simulink model "controller_ballcatcher_overdo"  (R2018b)
settings: Solver=FixedStepDiscrete  StartTime=0.0  StopTime=10.0  FixedStep=param_controller.T_a  RelTol=1e-3
InitFcn:
  | iiwa_joint_trajectoryfollowingcontrol_rigid_parameters;
values from neighbouring files (symbols this model uses):
  estimator_init_struct = struct()    [init_estimator_struct.m]
  filter_tau_p_slow_T_1 = filter_tau_slow_T_1    [parameters.m]
  filter_tau_p_T_1 = filter_tau_T_1    [parameters.m]
  filter_tau_slow_T_1 = 1./(2*pi*[200;200;200;200;200;200;200])    [parameters.m]
  filter_tau_T_1 = 1./(2*pi*[400;400;400;400;500;1000;1000])    [parameters.m]
  filter_theta_p_slow_T_1 = filter_tau_slow_T_1    [parameters.m]
  filter_theta_p_T_1 = filter_tau_T_1    [parameters.m]
  filter_theta_slow_T_1 = filter_tau_slow_T_1    [parameters.m]
  height_of_catch = 0.9    [init_estimator_struct.m]
  optitrack_data = struct()    [init_parabola.m]
  param_nullspace = struct()    [parameters.m]
  param_robot = struct()    [parameters.m]
  positions = struct()    [init_common_positions.m]
  sensor_torque_offset = [0.53;-0.095;-0.189;0.07;-0.058;0.0025;-0.12]    [parameters.m]
  timing = struct()    [parameters.m]
undefined symbols (not defined in the file or in its folder): param_controller
libraries: simulink_extras x1
(part 2 of 2)

== matlab function controller_ballcatcher_overdo/Chart1/estimate_parabola/Parabola Estimator ==
  data: t_in input; t_start input; point_in input; height_of_catch parameter; pd output; estimator_init_struct parameter; init input; pd_p output; use_pred output; t_catch_predict output; timing parameter; prediction_update output; init_number_of_samples input
function [pd,pd_p,use_pred,t_catch_predict,prediction_update] = fcn(t_in,t_start,point_in,height_of_catch,estimator_init_struct,init,timing,init_number_of_samples)

    t_for_est = t_in-t_start;
    t_move_start = timing.T_optitrack*init_number_of_samples;
    t_start_g = t_start + t_move_start;
    prediction_update = 0;
    
    persistent use_pred_p t_catch_predict_p t_zd;
    if init || isempty(t_catch_predict_p)
        use_pred_p = 0;
        t_catch_predict_p = [t_start_g,t_start_g+1];
        t_zd = t_move_start+0.5;
    end
    
    if t_in >= t_catch_predict_p(1) && t_in <= t_catch_predict_p(2)
        use_pred_p = 1;
        g = 9.81; 
        
        [estimations,prediction_update]=estimate_parabola(t_for_est,point_in,estimator_init_struct,init,timing);
        x0_est = estimations.x0_est;
        vx0_est = estimations.vx0_est;
        y0_est = estimations.y0_est;
        vy0_est = estimations.vy0_est;
        z0_est = estimations.z0_est;
        vz0_est = estimations.vz0_est;

        % parabola equations
        x = @(ti,x0_t,vx0_t) ( x0_t + vx0_t*ti );
        y = @(ti,y0_t,vy0_t) ( y0_t + vy0_t*ti );
        z = @(ti,z0_t,vz0_t) ( z0_t + vz0_t*ti - (g/2)*ti.^2 );

        % derivative equations
        x_p = @(vx0_t) ( vx0_t );
        y_p = @(vy0_t) ( vy0_t );
        z_p = @(ti,vz0_t) ( vz0_t - g*ti );

        % calculate time to catch
        za = -(g/2);
        zb = vz0_est;
        zc = z0_est;
        
        descriminant = -4*za*zc+4*za*height_of_catch+zb^2;
        if descriminant >= 0
           t_zd = -(zb+sqrt(descriminant))/(2*za);
        else
           fprintf('WARNING: Complex solution for catching time');
        end
        
        % calculate catch coordinates
        x_out = x(t_zd,x0_est,vx0_est);
        y_out = y(t_zd,y0_est,vy0_est);
        z_out = z(t_zd,z0_est,vz0_est);

        % calculate derivatives (for ee orientation)
        x_out_p = x_p(vx0_est);
        y_out_p = y_p(vy0_est);
        z_out_p = z_p(t_zd,vz0_est);
        
        t_catch_predict_p = [t_start_g,t_zd+t_start]; % -0.1 -> would be 100ms "time buffer"
    else
        use_pred_p = 0;
        [~]=estimate_parabola(t_for_est,point_in,estimator_init_struct,init,timing);
        
        x_out = 0;
        y_out = 0;
        z_out = 0;

        x_out_p = 0;
        y_out_p = 0;
        z_out_p = 0;
    end
    
    % set outputs
    use_pred = use_pred_p;
    t_catch_predict = t_catch_predict_p;
    
    pd = [x_out,y_out,z_out];
    pd_p = [x_out_p,y_out_p,z_out_p]*(-1); % *(-1) because we want the
    % endeffector z-axis to point towards the ball
end

== matlab function controller_ballcatcher_overdo/Trajectory Generation/Trajectory generator q ==
  data: start input; stop input; reset input; robot_model input; q_d output; q_target input; duration input; param_controller parameter
function q_d = fcn(start,stop,reset,robot_model,q_target,duration,param_controller)
  persistent last_start;
  persistent last_stop;
  persistent started;
  persistent q__0;
  persistent q__T;
  persistent t;
  persistent T;
  
  if(isempty(last_start))
    last_start=start;
  end
  if(isempty(last_stop))
    last_stop=stop;
  end
  if(isempty(started))
    started=0;
  end
  if(isempty(t))
    t=0;
  end
  if(isempty(q__0))
    q__0=robot_model.q;
  end
  if(isempty(q__T))
    q__T=q_target;
  end
  if(isempty(T))
    T=duration;
  end
  
  if(reset)
    q__0=robot_model.q;
    q__T=q_target;
    T=duration;
    started=0;
    t=0;
  else
    if(started==1 && last_stop~=stop && stop==1)
      started=0;
    elseif(started==0 && last_start~=start && start==1)
      started=1;
    end
  end
  last_start=start;
  last_stop=stop;
  
  if(t<=0)
    q_d=[q__0;zeros(size(q__0));zeros(size(q__0))];
  elseif(t>=T)
    q_d=[q__T;zeros(size(q__T));zeros(size(q__T))];
  else
    t1 = (q__0 - q__T);
    t2 = 1 / T;
    t3 = (t ^ 2);
    t4 = (t2 ^ 2);
    t5 = (t2 * t4 ^ 2);
    t6 = (t * t2);
    t7 = (t - T);
    q_d = [q__0 + t * t3 * t2 * t4 * t1 * (t6 * (-6 * t6 + 15) - 10);...
      -30 * t3 * t1 * t7 ^ 2 * t5;...
      60 * t * t1 * t7 * (T - 2 * t) * t5];
  end
  if(started==1)
    t=t+param_controller.T_a;
  else
    %Hold last position, set velocity and acceleration zero
    n=7;
    q_d(n+1:end)=0;
  end
end

== matlab function controller_ballcatcher_overdo/Friction Compensation/Friction Observer discrete ==
  settings: sampleTime=param.T_a
  data: motion_enabled input; tau_m input; tau input; tau_p input; theta_p input; tau_fm_hat output; param_robot parameter; L input; param_controller parameter; tau_f_model output; friction_model input
function [tau_fm_hat,tau_f_model]  = fcn(motion_enabled,tau_m,tau,tau_p,theta_p, param_robot,L, param_controller, friction_model)
  persistent x_theta_p_hat;
  
  T_a=param_controller.T_a;
  B=param_robot.B;

  if(isempty(x_theta_p_hat))
    x_theta_p_hat=zeros(param_robot.n,1);
  end
  
  if(motion_enabled)
    tau_c_plus=friction_model(1:param_robot.n);
    tau_c_minus=friction_model(param_robot.n+1:2*param_robot.n);
    E=friction_model(2*param_robot.n+1:3*param_robot.n);
    tau_v=friction_model(3*param_robot.n+1:4*param_robot.n);
    use_theta_p_hat=friction_model(4*param_robot.n+1);
    use_q_p=friction_model(4*param_robot.n+2);
    subtract_model=friction_model(4*param_robot.n+3);
    if(use_theta_p_hat)
      tmp=x_theta_p_hat;
    else
      tmp=theta_p;
    end
    if(use_q_p)
      q_p=tmp-param_robot.K\tau_p;
    else
      q_p=tmp;
    end
    %tau_f_model is the downforce friction, which cannot be observed, since
    %it happens after the torque sensor with respect to q_p.
    %This friction torque can be added to the motor torque to compensate for
    %this additional friction. It is _not_ subtracted from tau_m in the
    %friction observer, since it is additional torque, which has to appear
    %at the torque sensor and is required to overcome friction in the
    %downforce train.
    tau_f_model=zeros(size(q_p));
    c=q_p>=0;
    tau_f_model(c)=tau_c_plus(c).*tanh(E(c).*q_p(c));
    tau_f_model(~c)=tau_c_minus(~c).*tanh(E(~c).*q_p(~c));
    tau_f_model=tau_f_model+tau_v.*q_p;
    
    %Estimated, unmodeled friction
    tau_fm_hat=-L.*diag(param_robot.B).*(theta_p-x_theta_p_hat);
    %The term tau_m is the feedback torque from the motor. It contains the
    %added "tau_fm_hat", therefore it has to be subtracted, before feeding
    %it into the observer.
    %Notice, that not the actual control value is used, but the sensor
    %value from the motor. The latter signal is very, very noisy (standard
    %deviation of about 3 Nm at rest), but it shows the best behaviour for
    %estimating friction. It is also convenient, that the sensor value
    %implicitly contains the low-level saturation of the commanded value.
    if(subtract_model)
      x_theta_p_hat=x_theta_p_hat+T_a*(B\(tau_m-tau-tau_f_model-tau_fm_hat));
    else
      x_theta_p_hat=x_theta_p_hat+T_a*(B\(tau_m-tau-tau_fm_hat));
    end
  else
    x_theta_p_hat=zeros(param_robot.n,1);
    tau_fm_hat=zeros(param_robot.n,1);
    tau_f_model=zeros(param_robot.n,1);
  end
end

== matlab function controller_ballcatcher_overdo/Sensor Filters/f_theta_slow ==
  data: u input; theta_slow output; param_controller parameter; filter_theta_slow_T_1 parameter
function theta_slow = func(u,param_controller, filter_theta_slow_T_1)
  persistent x;
  
  T_1=filter_theta_slow_T_1;
  alpha=exp(-param_controller.T_a./T_1);
  if(isempty(x))
    x=1./(1-alpha).*u;
    theta_slow=u;
  else
    theta_slow=(1-alpha).*x;
    x=alpha.*x+u;
  end
end

== matlab function controller_ballcatcher_overdo/Sensor Filters/f_tau_p_slow ==
  data: u input; tau_p_slow output; filter_tau_p_slow_T_1 parameter; param_controller parameter
function tau_p_slow = func(u,filter_tau_p_slow_T_1,param_controller)
  persistent x;
  
  T_1=filter_tau_p_slow_T_1;
  V=1/param_controller.T_a*(1-exp(-param_controller.T_a./T_1));
  if(isempty(x))
    x=-V.*u;
    tau_p_slow=zeros(size(u));
  else
    tau_p_slow=x+V.*u;
    x=exp(-param_controller.T_a./T_1).*x+(exp(-param_controller.T_a./T_1)-1).*V.*u;
  end
end

== matlab function controller_ballcatcher_overdo/Sensor Filters/f_theta_p_slow ==
  data: u input; theta_p_slow output; filter_theta_p_slow_T_1 parameter; param_controller parameter
function theta_p_slow = func(u,filter_theta_p_slow_T_1,param_controller)
  persistent x;
  
  T_1=filter_theta_p_slow_T_1;
  V=1/param_controller.T_a*(1-exp(-param_controller.T_a./T_1));
  if(isempty(x))
    x=-V.*u;
    theta_p_slow=zeros(size(u));
  else
    theta_p_slow=x+V.*u;
    x=exp(-param_controller.T_a./T_1).*x+(exp(-param_controller.T_a./T_1)-1).*V.*u;
  end
end

== matlab function controller_ballcatcher_overdo/Rigid Body Controller/Controller Enable ==
  data: enable1 output; enable2 output; enable3 output; enable4 output; enable5 output; enable6 output; enable7 output; enable8 output; selector input uint32; enable9 output; enable10 output
function [enable1,enable2,enable3,enable4,enable5,enable6,enable7,enable8,enable9,enable10] = fcn(selector)
    enable1=(selector==1);
    enable2=(selector==2);
    enable3=(selector==3);
    enable4=(selector==4);
    enable5=(selector==5);
    enable6=(selector==6);
    enable7=(selector==7);
    enable8=(selector==8);
    enable9=(selector==9);
    enable10=(selector==10);
end

== matlab function controller_ballcatcher_overdo/Rigid Body Controller/Controller Selector ==
  data: selector input uint32; input1 input; input2 input; input3 input; input4 input; input5 input; input6 input; input7 input; input8 input; output output; input9 input; input10 input
function output = fcn(selector,input1,input2,input3,input4,input5,input6,input7,input8,input9,input10)
    switch selector
        case 1
            output=input1;
        case 2
            output=input2;
        case 3
            output=input3;
        case 4
            output=input4;
        case 5
            output=input5;
        case 6
            output=input6;
        case 7
            output=input7;
        case 8
            output=input8;
        case 9
            output=input9;
        case 10
            output=input10;
        otherwise
            output=zeros(size(input1));
    end
end
